simulink model "FSK"  (R2014a)
settings: Solver=ode45  StartTime=0.0  StopTime=10.0  RelTol=1e-3
settings Model: Creator=admin  LastModifiedBy=admin

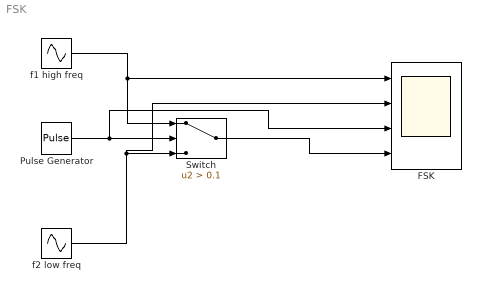
== system FSK ==
  FSK : Scope  NumInputPorts=4
      settings: YMin=-5~-5~-5~-5  YMax=5~5~5~5
  Pulse Generator : DiscretePulseGenerator  PulseType=Time based  Amplitude=4  PulseWidth=50
  Switch : Switch  Criteria=u2 > Threshold  Threshold=0.1
  f1 high freq : Sin  Amplitude=4  Frequency=50  SampleTime=0.001
  f2 low freq : Sin  Amplitude=4  Frequency=30  SampleTime=0.001
  wires:
  Pulse Generator/1 -> FSK/3, Switch/2
  f1 high freq/1 -> FSK/1, Switch/1
  f2 low freq/1 -> FSK/2, Switch/3
  Switch/1 -> FSK/4
